simulink model "LR4_MostKran_1"  (R2015b)
settings: Solver=FixedStepAuto  StartTime=0.0  StopTime=300.0  FixedStep=dT  RelTol=1e-3
values from neighbouring files (symbols this model uses):
  A = [0, 1, 0, 0;  0, 0, a23, 0;  0, 0, 0, 1;  0, 0, a43, 0]    [LR_4_MostKran.m]
  B = [0; b2; 0; b4]    [LR_4_MostKran.m]
  C = [1, 0, 0, 0; 0, 1, 0, 0; 0, 0, 1, 0; 0, 0, 0, 1]    [LR_4_MostKran.m]
  D = [0; 0; 0; 0]    [LR_4_MostKran.m]
  fisREG = readfis('RgMostKran_1')    [LR_4_MostKran.m]
  KdE = 1/6    (= 0.166666666667)    [LR_4_MostKran.m]
  KEr = 1/80    (= 0.0125)    [LR_4_MostKran.m]
  KU = 20    [LR_4_MostKran.m]
  X0 = [0; 0; 0; 0]    [LR_4_MostKran.m]
undefined symbols (not defined in the file or in its folder): sigbuilder_block
libraries: fuzblock x1
settings Model: Creator=Сергей  LastModifiedBy=Сергей

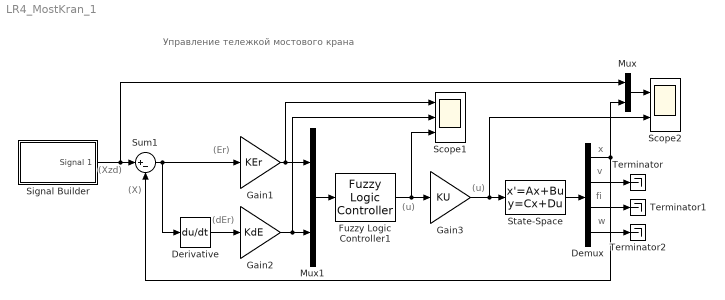
== system LR4_MostKran_1 ==
  note: w
  note: fi
  note: v
  note: x
  note: (Xzd)
  note: Управление тележкой мостового крана
  note: (Er)
  note: (dEr)
  note: (u)
  note: (u)
  note: (X)
  Demux : Demux
  Derivative : Derivative
  Fuzzy Logic Controller1 : fuzblock/Fuzzy Logic  Controller  fis=[fisREG]
  Gain1 : Gain  Gain=KEr
  Gain2 : Gain  Gain=KdE
  Gain3 : Gain  Gain=KU
  Mux : Mux  Inputs=2
  Mux1 : Mux  Inputs=2
  Scope1 : Scope  NumInputPorts=3
  Scope2 : Scope  NumInputPorts=2
  Signal Builder : Subsystem  Tag=STV Subsys  LoadFcn=sigbuilder_block('load');  StartFcn=sigbuilder_block('start');  StopFcn=sigbuilder_block('stop');  ClipboardFcn=sigbuilder_block('clipboard');  mask(Sigbuilder block){}
      mask help: Simulink:masks:SigbuilderBlock_MD
      mask init:
      | if ~strcmp(get_param(bdroot(gcbh),'SimulationStatus'),'stopped') tuvar = sigbuilder_block('maskInit'); end
      settings: CopyFcn=sigbuilder_block('copy');  DeleteFcn=sigbuilder_block('delete');  ModelCloseFcn=sigbuilder_block('modelClose');  PreSaveFcn=sigbuilder_block('preSave');  PauseFcn=sigbuilder_block('pause');  ContinueFcn=sigbuilder_block('continue');  NameChangeFcn=sigbuilder_block('namechange');  OpenFcn=sigbuilder_block('open',[63.75 114.75 550.5 399.75 ]);  CloseFcn=sigbuilder_block('close');
      mask Display: plot(0, 0, 100, 100,[2, 2, 32, 32, 2], [68, 8, 8, 68, 68],[32, 2], [38, 38], [32, 19, 2],[53, 60, 44], [32, 17, 17, 2],[16, 16, 31, 31]);txt = getActiveGroup(gcbh);text(2, 100, txt,'verticalAlignment', 'top');
  State-Space : StateSpace  A=A  B=B  C=C  D=D  X0=X0
  Sum1 : Sum  Inputs=|+-
  Terminator : Terminator
  Terminator1 : Terminator
  Terminator2 : Terminator
  wires:
  Signal Builder/1(Signal 1) -> Mux/1, Sum1/1
  State-Space/1 -> Demux/1
  Demux/1 -> Sum1/2, Mux/2
  Demux/2 -> Terminator/1
  Demux/3 -> Terminator1/1
  Demux/4 -> Terminator2/1
  Mux1/1 -> Fuzzy Logic Controller1/1
  Sum1/1 -> Derivative/1, Gain1/1
  Gain1/1 -> Scope1/1, Mux1/1
  Gain2/1 -> Scope1/2, Mux1/2
  Mux/1 -> Scope2/1
  Fuzzy Logic Controller1/1 -> Gain3/1, Scope1/3
  Gain3/1 -> Scope2/2, State-Space/1
  Derivative/1 -> Gain2/1

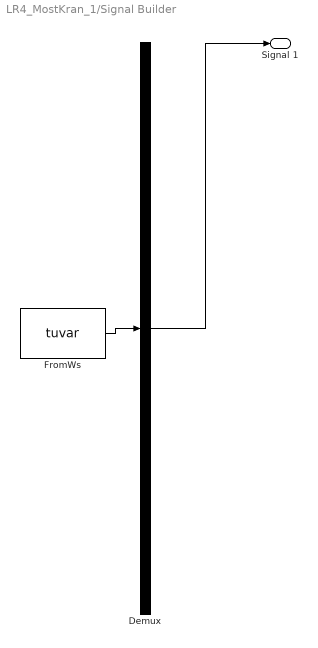
== system LR4_MostKran_1/Signal Builder ==
  Demux : Demux  Tag=STV Demux  Outputs=1
  FromWs : FromWorkspace  Tag=STV FromWs  VariableName=tuvar  SampleTime=0
      SigBuilderData=|
      | common.afterFinalStr = 'Extrapolate'
      | common.sampleTime = 0
      | dataSet.timeRange = [0 300]
      | dataSet.name = 'Group 1'
      | sbobj.Groups.Name = 'Group 1'
      | sbobj.Groups.Signals.Name = 'Signal 1'
      | sbobj.Groups.Signals.XData = [0 10 10 100 100 200 200 300]
      | sbobj.Groups.Signals.YData = [0 0 40 40 20 20 -0.2 -0.2]
      | sbobj.Groups.TimeRange = [0 300]
  Signal 1 : Outport  Tag=STV Outport
  wires:
  Demux/1 -> Signal 1/1
  FromWs/1 -> Demux/1
